simulink model "b747_lqr"  (R2025b)
settings: Solver=VariableStepAuto  StartTime=0.0  StopTime=T_end  RelTol=1e-3
undefined symbols (not defined in the file): A, B, K_lqr, N_bar
libraries: simulink_extras x9
settings Model: Creator=User  LastModifiedBy=User
settings DataIOCC: ReturnWorkspaceOutputsName=out_lqr

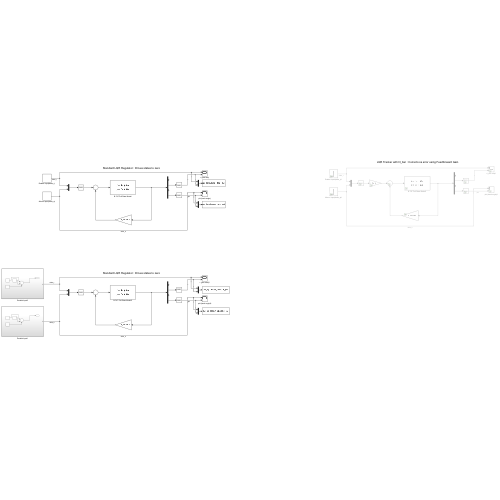
[thumbnail: Simulink's stored preview of the top-level diagram]
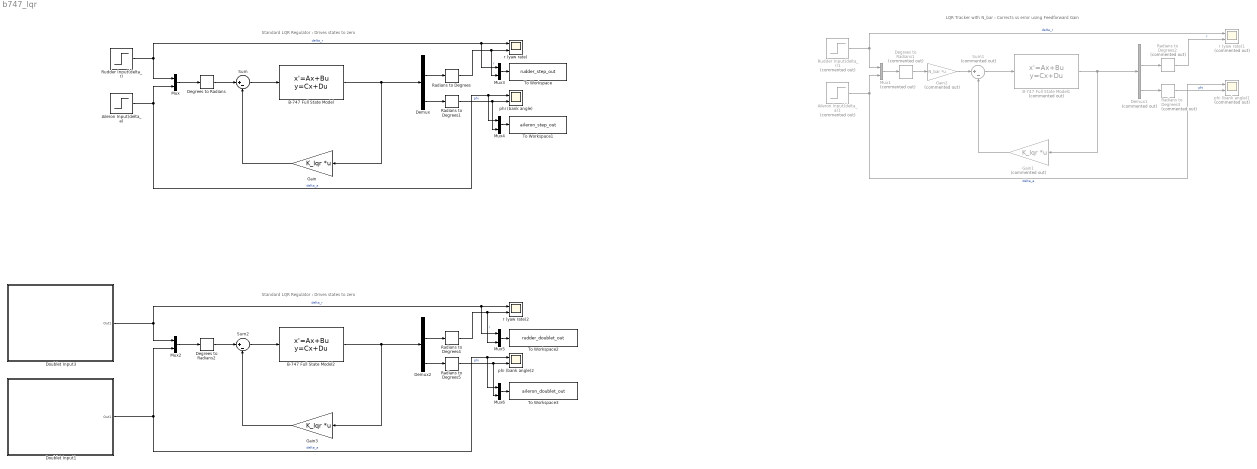
== system b747_lqr ==
  note: Standard LQR Regulator : Drives states to zero
  note: LQR Tracker with N_bar : Corrects ss error using Feedforward Gain
  note: Standard LQR Regulator : Drives states to zero
  Aileron Input(delta_a) : Step  SampleTime=0
  Aileron Input(delta_a)1 : Step  Commented=on  SampleTime=0
  B-747 Full State Model : StateSpace  A=A  B=B  C=eye(4)  D=zeros(4,2)  InitialCondition=0
  B-747 Full State Model1 : StateSpace  Commented=on  A=A  B=B  C=eye(4)  D=zeros(4,2)  InitialCondition=0
  B-747 Full State Model2 : StateSpace  A=A  B=B  C=eye(4)  D=zeros(4,2)  InitialCondition=0
  Degrees to Radians : simulink_extras/Transformations/Degrees to Radians
  Degrees to Radians1 : simulink_extras/Transformations/Degrees to Radians  Commented=on
  Degrees to Radians2 : simulink_extras/Transformations/Degrees to Radians
  Demux : Demux
  Demux1 : Demux  Commented=on
  Demux2 : Demux
  Doublet Input1 : Subsystem
  Doublet Input3 : Subsystem
  Gain : Gain  Gain=K_lqr  Multiplication=Matrix(K*u) (u vector)
  Gain1 : Gain  Commented=on  Gain=K_lqr  Multiplication=Matrix(K*u) (u vector)
  Gain2 : Gain  Commented=on  Gain=N_bar  Multiplication=Matrix(K*u)
  Gain3 : Gain  Gain=K_lqr  Multiplication=Matrix(K*u) (u vector)
  Mux{,2..6} (6 alike) : Mux  Inputs=2
  Mux1 : Mux  Commented=on  Inputs=2
  Radians to Degrees{,1,4..5} (4 alike) : simulink_extras/Transformations/Radians to Degrees
  Radians to Degrees2 : simulink_extras/Transformations/Radians to Degrees  Commented=on
  Radians to Degrees3 : simulink_extras/Transformations/Radians to Degrees  Commented=on
  Rudder Input(delta_r) : Step  SampleTime=0
  Rudder Input(delta_r)1 : Step  Commented=on  SampleTime=0
  Sum : Sum  Inputs=|+-
  Sum1 : Sum  Commented=on  Inputs=|+-
  Sum2 : Sum  Inputs=|+-
  To Workspace : ToWorkspace  VariableName=rudder_step_out  SaveFormat=Timeseries  SampleTime=-1
  To Workspace1 : ToWorkspace  VariableName=aileron_step_out  SaveFormat=Timeseries  SampleTime=-1
  To Workspace2 : ToWorkspace  VariableName=rudder_doublet_out  SaveFormat=Timeseries  SampleTime=-1
  To Workspace3 : ToWorkspace  VariableName=aileron_doublet_out  SaveFormat=Timeseries  SampleTime=-1
  phi (bank angle) : Scope  NumInputPorts=2
      settings: ActiveDisplayYMinimum=-2.3810081471479183  ActiveDisplayYMaximum=2.8692007195081346
  phi (bank angle)1 : Scope  Commented=on  NumInputPorts=2
      settings: ActiveDisplayYMinimum=-44.072090994045865  ActiveDisplayYMaximum=20.435040293487692  DataLoggingVariableName=ScopeData2
  phi (bank angle)2 : Scope  NumInputPorts=2
      settings: ActiveDisplayYMinimum=-1.8883616484098997  ActiveDisplayYMaximum=2.2253143780398288  DataLoggingVariableName=ScopeData4
  r (yaw rate) : Scope  NumInputPorts=2
      settings: ActiveDisplayYMinimum=-3.190844085859831  ActiveDisplayYMaximum=5.1579890290854173
  r (yaw rate)1 : Scope  Commented=on  NumInputPorts=2
      settings: ActiveDisplayYMinimum=-13.751312438921728  ActiveDisplayYMaximum=24.136021964748458  DataLoggingVariableName=ScopeData3
  r (yaw rate)2 : Scope  NumInputPorts=2
      settings: ActiveDisplayYMinimum=-4.0337819411933076  ActiveDisplayYMaximum=5.6310359934951872  DataLoggingVariableName=ScopeData5
  wires:
  Rudder Input(delta_r)/1 -> Mux3/1, r (yaw rate)/1, Mux/1  "delta_r"
  Aileron Input(delta_a)/1 -> Mux4/1, phi (bank angle)/1, Mux/2  "delta_a"
  B-747 Full State Model/1 -> Gain/1, Demux/1
  Demux/2 -> Radians to Degrees/1
  Radians to Degrees/1 -> Mux3/2, r (yaw rate)/2  "r"
  Demux/4 -> Radians to Degrees1/1
  Radians to Degrees1/1 -> Mux4/2, phi (bank angle)/2  "phi"
  Mux/1 -> Degrees to Radians/1
  Degrees to Radians/1 -> Sum/1
  Sum/1 -> B-747 Full State Model/1
  Gain/1 -> Sum/2
  Aileron Input(delta_a)1/1 -> phi (bank angle)1/1, Mux1/2  "delta_a"
  Radians to Degrees3/1 -> phi (bank angle)1/2  "phi"
  Gain1/1 -> Sum1/2
  Rudder Input(delta_r)1/1 -> r (yaw rate)1/1, Mux1/1  "delta_r"
  Demux1/4 -> Radians to Degrees3/1
  B-747 Full State Model1/1 -> Gain1/1, Demux1/1
  Mux1/1 -> Degrees to Radians1/1
  Sum1/1 -> B-747 Full State Model1/1
  Radians to Degrees2/1 -> r (yaw rate)1/2  "r"
  Demux1/2 -> Radians to Degrees2/1
  Degrees to Radians1/1 -> Gain2/1
  Gain2/1 -> Sum1/1
  Mux2/1 -> Degrees to Radians2/1
  Degrees to Radians2/1 -> Sum2/1
  Radians to Degrees4/1 -> Mux5/2, r (yaw rate)2/2  "r"
  B-747 Full State Model2/1 -> Gain3/1, Demux2/1
  Gain3/1 -> Sum2/2
  Demux2/4 -> Radians to Degrees5/1
  Doublet Input3/1(Out1) -> Mux5/1, r (yaw rate)2/1, Mux2/1  "delta_r"
  Demux2/2 -> Radians to Degrees4/1
  Radians to Degrees5/1 -> Mux6/2, phi (bank angle)2/2  "phi"
  Sum2/1 -> B-747 Full State Model2/1
  Doublet Input1/1(Out1) -> Mux6/1, phi (bank angle)2/1, Mux2/2  "delta_a"
  Mux3/1 -> To Workspace/1
  Mux4/1 -> To Workspace1/1
  Mux5/1 -> To Workspace2/1
  Mux6/1 -> To Workspace3/1

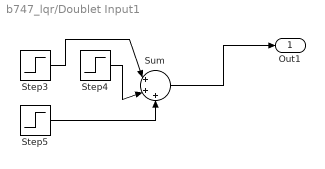
== system b747_lqr/Doublet Input1 ==
  Step3 : Step  Time=2  After=-2  SampleTime=0
  Step4 : Step  SampleTime=0
  Step5 : Step  Time=3  SampleTime=0
  Sum : Sum  Inputs=|+++
  Out1 : Outport
  wires:
  Step4/1 -> Sum/2
  Step5/1 -> Sum/3
  Step3/1 -> Sum/1
  Sum/1 -> Out1/1

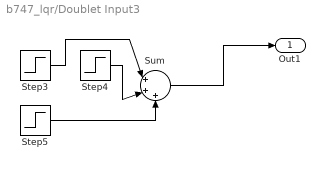
== system b747_lqr/Doublet Input3 ==
  Step3 : Step  Time=2  After=-2  SampleTime=0
  Step4 : Step  SampleTime=0
  Step5 : Step  Time=3  SampleTime=0
  Sum : Sum  Inputs=|+++
  Out1 : Outport
  wires:
  Step4/1 -> Sum/2
  Step5/1 -> Sum/3
  Step3/1 -> Sum/1
  Sum/1 -> Out1/1
